simulink model "STATCOM"  (R2024a)
settings: Solver=FixedStepDiscrete  StartTime=0.0  StopTime=0.4  FixedStep=Ts  RelTol=1e-3
InitFcn:
  | Ts=25e-6;
  | xInitial = STATCOMInit;
undefined symbols (not defined in the file or in its folder): DiscIntNeverNeededParam
libraries: spsThreeLevelBridgeLib x4, spsVoltageMeasurementLib x4, spsZigzagPhaseShiftingTransformerLib x4, spsThreePhaseVIMeasurementLib x3, spsDistributedParametersLineLib x3, spsSecondOrderFilterLib x3, spsSeriesRLCBranchLib x2, spsThreePhaseSourceLib x2, spsGroundLib x2, spsabctodq0Lib x2, spsThreePhaseSeriesRLCLoadLib x1, spsThreePhaseParallelRLCLoadLib x1
(part 2 of 3)

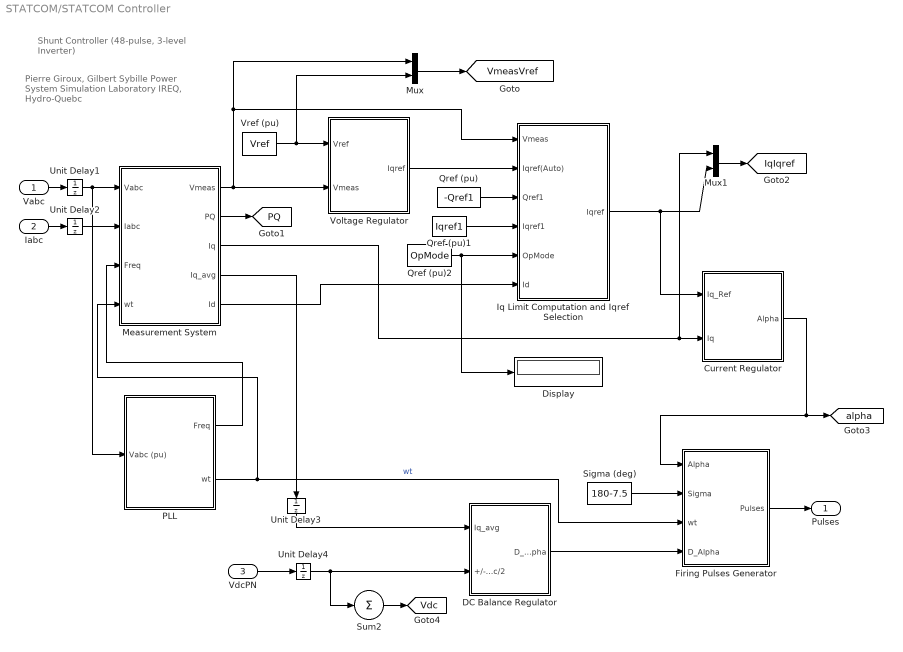
== system STATCOM/STATCOM Controller ==
  note: Pierre Giroux, Gilbert Sybille
      | Power System Simulation Laboratory
      | IREQ, Hydro-Quebc
  note: Shunt Controller
      | (48-pulse, 3-level Inverter)
  Vabc : Inport  PortDimensions=3
  Iabc : Inport  Port=2  PortDimensions=3
  VdcPN : Inport  Port=3  PortDimensions=2
  Current Regulator : Subsystem  mask(Discrete PI Controller){Kp=Kp_I, Ki=Ki_I, Par_Limits=[80 -80], Init=0, Ts=Ts}
      mask prompts: Kp "Proportional gain (Kp):"; Ki "Integral gain (Ki):"; Par_Limits "Output limits: [ Upper   Lower ]"; Init "Output initial value:"; Ts "Sample time:"
      mask help: This block implements a discrete PI controller.
      mask init:
      | UpperLimit=Par_Limits(1);
      | LowerLimit=Par_Limits(2);
  DC Balance Regulator : Subsystem
  Display : Display
  Firing Pulses Generator : Subsystem
  Iq Limit Computation and Iqref Selection : Subsystem
  Measurement System : Subsystem
  Mux : Mux  Inputs=2
  Mux1 : Mux  Inputs=2
  PLL : Subsystem  mask(Discrete 3-phase PLL){Nstep=1, Par_Init=[0 60], ParK=[60 1400], Ts=Ts}
      mask prompts: Nstep "PLL timing correction (in number of time step)"; Par_Init "Initial inputs:[ Phase(degrees)   Frequency(Hz) ]"; ParK "Regulator gains [ Kp  Ki ]"; Ts "Sample time:"
      mask help:
      | This Phase Locked Loop (PLL) system can be used  to synchronize on a set of variable frequency, three-phase sinusoidal signals.
      |
      | Input 1: Vector containing the normalized
      |              three-phase signals [Va Vb Vc]
      | Output 1:  Measured frequency (Hz) = w/(2pi)
      | Output 2:  Ramp w.t   varying between  0 and 2*pi,
      | synchronized on zero crossings of the fundamental (positive-sequence) of phase A.
      | Output 3: Vector [sin(wt) cos(wt)]
      mask init:
      | Kp=ParK(1);
      | Ki=ParK(2);
      | Phase_Init=Par_Init(1);
      | Finit=Par_Init(2);
  Qref (pu) : Constant  Value=-Qref1
  Qref (pu)1 : Constant  Value=Iqref1
  Qref (pu)2 : Constant  Value=OpMode
  Sigma (deg) : Constant  Value=180-7.5
  Sum2 : Sum  Inputs=1  InputSameDT=on  SaturateOnIntegerOverflow=on  OutDataTypeStr=Inherit: Same as first input
  Unit Delay{1..4} (4 alike) : UnitDelay  SampleTime=Ts  HasFrameUpgradeWarning=on
  Voltage Regulator : Subsystem  mask(Discrete PI Controller){Droop=Droop, Kp=Kp_V, Ki=Ki_V, Par_Limits=[1 -1], Init=0, Ts=Ts}
      mask prompts: Droop "Droop (pu/100MVA):"; Kp "Proportional gain (Kp):"; Ki "Integral gain (Ki):"; Par_Limits "Output limits: [ Upper   Lower ]"; Init "Output initial value:"; Ts "Sample time:"
      mask help: This block implements a discrete PI controller.
      mask init:
      | UpperLimit=Par_Limits(1);
      | LowerLimit=Par_Limits(2);
  Vref (pu) : Constant  Value=Vref
  Pulses : Outport  VectorParamsAs1DForOutWhenUnconnected=off
  tag scope: IqIqref=global, PQ=global, Vdc=global, VmeasVref=global, alpha=global
  wires:
  DC Balance Regulator/1(D_Alpha) -> Firing Pulses Generator/4(D_Alpha)
  Unit Delay4/1 -> Sum2/1, DC Balance Regulator/2(+/-Vdc/2)
  Unit Delay2/1 -> Measurement System/2(Iabc)
  Unit Delay1/1 -> Measurement System/1(Vabc), PLL/1(Vabc (pu))
  Sum2/1 -> [Vdc]
  Iabc/1 -> Unit Delay2/1
  Firing Pulses Generator/1(Pulses) -> Pulses/1
  VdcPN/1 -> Unit Delay4/1
  Mux/1 -> [VmeasVref]
  Unit Delay3/1 -> DC Balance Regulator/1(Iq_avg)
  Measurement System/4(Iq_avg) -> Unit Delay3/1
  Vabc/1 -> Unit Delay1/1
  PLL/2(wt) -> Measurement System/4(wt), Firing Pulses Generator/3(wt)  "wt"
  PLL/1(Freq) -> Measurement System/3(Freq)
  Qref (pu)2/1 -> Display/1, Iq Limit Computation and Iqref Selection/5(OpMode)
  Voltage Regulator/1(Iqref) -> Iq Limit Computation and Iqref Selection/2(Iqref(Auto))
  Measurement System/2(PQ) -> [PQ]
  Measurement System/1(Vmeas) -> Mux/1, Iq Limit Computation and Iqref Selection/1(Vmeas), Voltage Regulator/2(Vmeas)
  Qref (pu)/1 -> Iq Limit Computation and Iqref Selection/3(Qref1)
  Qref (pu)1/1 -> Iq Limit Computation and Iqref Selection/4(Iqref1)
  Measurement System/3(Iq) -> Current Regulator/2(Iq), Mux1/1
  Measurement System/5(Id) -> Iq Limit Computation and Iqref Selection/6(Id)
  Vref (pu)/1 -> Voltage Regulator/1(Vref), Mux/2
  Iq Limit Computation and Iqref Selection/1(Iqref) -> Current Regulator/1(Iq_Ref), Mux1/2
  Mux1/1 -> [IqIqref]
  Sigma (deg)/1 -> Firing Pulses Generator/2(Sigma)
  Current Regulator/1(Alpha) -> Firing Pulses Generator/1(Alpha), [alpha]

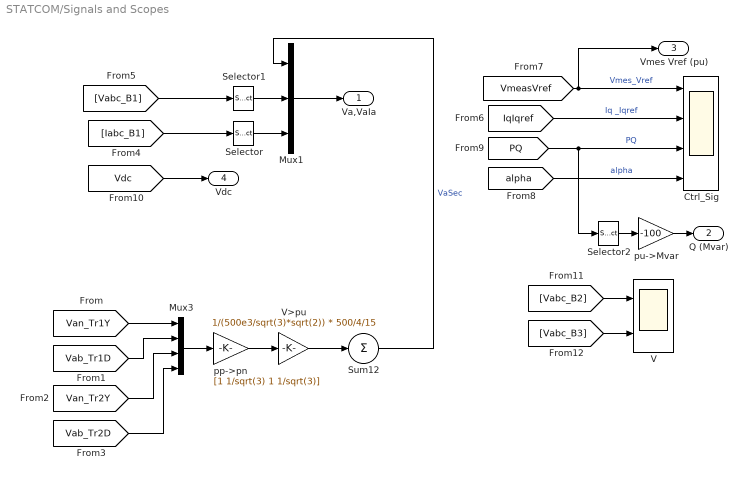
== system STATCOM/Signals and Scopes ==
  Ctrl_Sig : Scope  NumInputPorts=4
  Mux1 : Mux  Inputs=3
  Mux3 : Mux
  Selector : Selector  InputPortWidth=3  IndexOptions=Index vector (dialog)  Indices=1  OutputSizes=1
  Selector1 : Selector  InputPortWidth=3  IndexOptions=Index vector (dialog)  Indices=1  OutputSizes=1
  Selector2 : Selector  InputPortWidth=2  IndexOptions=Index vector (dialog)  Indices=2  OutputSizes=1
  Sum12 : Sum  Inputs=1  InputSameDT=on  SaturateOnIntegerOverflow=on  OutDataTypeStr=Inherit: Same as first input
  V : Scope  NumInputPorts=2
  "V>pu " : Gain  Gain=1/(500e3/sqrt(3)*sqrt(2)) * 500/4/15  SaturateOnIntegerOverflow=on  OutDataTypeStr=Inherit: Same as input  ParamDataTypeStr=Inherit: Same as input
  pp->pn : Gain  Gain=[1 1/sqrt(3) 1 1/sqrt(3)]  SaturateOnIntegerOverflow=on  OutDataTypeStr=Inherit: Same as input  ParamDataTypeStr=Inherit: Same as input
  pu->Mvar : Gain  Gain=-100  SaturateOnIntegerOverflow=on  OutDataTypeStr=Inherit: Same as input  ParamDataTypeStr=Inherit: Same as input
  Va,VaIa : Outport  VectorParamsAs1DForOutWhenUnconnected=off
  "Q (Mvar) " : Outport  Port=2  VectorParamsAs1DForOutWhenUnconnected=off
  Vmes Vref (pu) : Outport  Port=3  VectorParamsAs1DForOutWhenUnconnected=off
  Vdc : Outport  Port=4  VectorParamsAs1DForOutWhenUnconnected=off
  wires:
  "V>pu "/1 -> Sum12/1
  pp->pn/1 -> "V>pu "/1
  Mux3/1 -> pp->pn/1
  [Van_Tr1Y] -> Mux3/1
  [Vab_Tr1D] -> Mux3/2
  [Van_Tr2Y] -> Mux3/3
  [Vab_Tr2D] -> Mux3/4
  Mux1/1 -> Va,VaIa/1
  [VmeasVref] -> Vmes Vref (pu)/1, Ctrl_Sig/1  "Vmes_Vref"
  Selector1/1 -> Mux1/2
  Selector/1 -> Mux1/3
  Sum12/1 -> Mux1/1  "VaSec"
  [IqIqref] -> Ctrl_Sig/2  "Iq _Iqref"
  [PQ] -> Ctrl_Sig/3, Selector2/1  "PQ"
  [alpha] -> Ctrl_Sig/4  "alpha"
  [Vabc_B1] -> Selector1/1
  [Iabc_B1] -> Selector/1
  [Vdc] -> Vdc/1
  [Vabc_B2] -> V/1
  [Vabc_B3] -> V/2
  Selector2/1 -> pu->Mvar/1
  pu->Mvar/1 -> "Q (Mvar) "/1

== system STATCOM/STATCOM Controller/Current Regulator ==
  Iq_Ref : Inport
  Iq : Inport  Port=2
  Discrete-Time Integrator : DiscreteIntegrator  InitialCondition=Init  SampleTime=Ts  LimitOutput=on  UpperSaturationLimit=UpperLimit*10  LowerSaturationLimit=LowerLimit*10  ICPrevOutput=DiscIntNeverNeededParam  ICPrevScaledInput=DiscIntNeverNeededParam
  Kp4 : Gain  Gain=Kp  SaturateOnIntegerOverflow=on  OutDataTypeStr=Inherit: Same as input  ParamDataTypeStr=Inherit: Same as input
  Kp5 : Gain  Gain=Ki  SaturateOnIntegerOverflow=on  OutDataTypeStr=Inherit: Same as input  ParamDataTypeStr=Inherit: Same as input
  Saturation2 : Saturate  UpperLimit=UpperLimit  LowerLimit=LowerLimit
  Sum : Sum  Inputs=-+|  InputSameDT=on  SaturateOnIntegerOverflow=on  OutDataTypeStr=Inherit: Same as first input
  Sum6 : Sum  InputSameDT=on  SaturateOnIntegerOverflow=on  OutDataTypeStr=Inherit: Same as first input
  Alpha : Outport  InitialOutput=0  VectorParamsAs1DForOutWhenUnconnected=off
  wires:
  Sum/1 -> Kp4/1, Kp5/1  "Err"
  Iq/1 -> Sum/2
  Saturation2/1 -> Alpha/1
  Discrete-Time Integrator/1 -> Sum6/2
  Kp4/1 -> Sum6/1
  Kp5/1 -> Discrete-Time Integrator/1
  Sum6/1 -> Saturation2/1
  Iq_Ref/1 -> Sum/1

== system STATCOM/STATCOM Controller/DC Balance Regulator ==
  Iq_avg : Inport  PortDimensions=1
  +/-Vdc/2 : Inport  Port=2  PortDimensions=2
  " Mean value" : Subsystem  mask(Discrete Mean value){Freq=60, Vinit=0, Ts=Ts}
      mask prompts: Freq "Fundamental frequency (Hz):"; Vinit "Initial input (DC component):"; Ts "Sample time:"
      mask help:
      | This block computes the mean value of the input signal over a running window of one cycle of the specified fundamental frequency.
      | For the first cycle of simulation, the output is held constant to the value specified by the parameter "Initial input".
      mask init:
      | SamplesPerCycle=1/Freq/Ts;
      | RoundSamplesPerCycle=round(SamplesPerCycle);
      | Delay=RoundSamplesPerCycle*Ts - Ts/2;
      | Correction=SamplesPerCycle/RoundSamplesPerCycle - 1;
  Abs : Abs
  D_Alpha(Manual) : Constant  Value=0
  D_Alpha1 : Constant  Value=0
  D_Alpha2 : Constant  Value=0
  D_Alpha5 : Constant  Value=0.1
  Demux : Demux  Outputs=2
      settings: DisplayOption=none
  Gain : Gain  Gain=0  SaturateOnIntegerOverflow=on  OutDataTypeStr=Inherit: Same as input  ParamDataTypeStr=Inherit: Same as input
  Gain1 : Gain  Gain=-1  SaturateOnIntegerOverflow=on  OutDataTypeStr=Inherit: Same as input  ParamDataTypeStr=Inherit: Same as input
  Mode : Constant
  Multiport Switch : MultiPortSwitch
  PI Regulator : Subsystem  mask(Discrete PI Controller){Kp=0.001, Ki=0.01, Par_Limits=[2 -2], Init=0, Ts=Ts}
      mask prompts: Kp "Proportional gain (Kp):"; Ki "Integral gain (Ki):"; Par_Limits "Output limits: [ Upper   Lower ]"; Init "Output initial value:"; Ts "Sample time:"
      mask help: This block implements a discrete PI controller.
      mask init:
      | UpperLimit=Par_Limits(1);
      | LowerLimit=Par_Limits(2);
      mask Display: disp('PI');
  Relational Operator : RelationalOperator  Operator=<=
  Relational Operator1 : RelationalOperator  Operator=<
  Sum2 : Sum  Inputs=-+  InputSameDT=on  SaturateOnIntegerOverflow=on  OutDataTypeStr=Inherit: Same as first input
  Switch : Switch  Threshold=0.5
  Switch1 : Switch  Threshold=0.5
  D_Alpha : Outport  VectorParamsAs1DForOutWhenUnconnected=off
  wires:
  Demux/2 -> Sum2/2
  Demux/1 -> Sum2/1
  +/-Vdc/2/1 -> Demux/1
  Iq_avg/1 -> Relational Operator/1, Abs/1
  Sum2/1 -> " Mean value"/1(In)
  Switch1/1 -> PI Regulator/1(Error)
  Gain/1 -> Switch1/1
  " Mean value"/1(Mean) -> Gain/1, Switch1/3
  D_Alpha1/1 -> Relational Operator/2
  Abs/1 -> Relational Operator1/1
  D_Alpha5/1 -> Relational Operator1/2
  Gain1/1 -> Switch/3
  Relational Operator/1 -> Switch/2
  Switch/1 -> Multiport Switch/2  "Auto"
  D_Alpha2/1 -> Multiport Switch/4  "Off"
  Mode/1 -> Multiport Switch/1
  PI Regulator/1(Out) -> Switch/1, Gain1/1
  D_Alpha(Manual)/1 -> Multiport Switch/3  "Man"
  Multiport Switch/1 -> D_Alpha/1
  Relational Operator1/1 -> Switch1/2, PI Regulator/2(Reset)

== system STATCOM/STATCOM Controller/Firing Pulses Generator ==
  Alpha : Inport  PortDimensions=1
  Sigma : Inport  Port=2  PortDimensions=1
  wt : Inport  Port=3  PortDimensions=1
  D_Alpha : Inport  Port=4  PortDimensions=1
  " Deg->Rad" : Gain  Gain=pi/180  SaturateOnIntegerOverflow=on  OutDataTypeStr=Inherit: Same as input  ParamDataTypeStr=Inherit: Same as input
  Bridge 1D : Subsystem
  "Bridge 1Y " : Subsystem
  Bridge 2D : Subsystem
  Bridge 2Y : Subsystem
  Constant : Constant  Value=[0 -30 -15 -45]*pi/180 + 7.5*pi/180
  Deg->Rad : Gain  Gain=pi/180  SaturateOnIntegerOverflow=on  OutDataTypeStr=Inherit: Same as input  ParamDataTypeStr=Inherit: Same as input
  "Deg->Rad " : Gain  Gain=pi/180  SaturateOnIntegerOverflow=on  OutDataTypeStr=Inherit: Same as input  ParamDataTypeStr=Inherit: Same as input
  Demux : Demux
      settings: DisplayOption=none
  Mux : Mux  Inputs=[12 12 12 12]
  Sum : Sum  InputSameDT=on  SaturateOnIntegerOverflow=on  OutDataTypeStr=Inherit: Same as first input
  Pulses : Outport  VectorParamsAs1DForOutWhenUnconnected=off
  wires:
  Alpha/1 -> Deg->Rad/1
  Constant/1 -> Sum/2
  Sum/1 -> Demux/1
  "Bridge 1Y "/1(Pulses) -> Mux/1
  Mux/1 -> Pulses/1
  Demux/1 -> "Bridge 1Y "/1(wt)
  Sigma/1 -> "Deg->Rad "/1
  Demux/2 -> Bridge 1D/1(wt)
  Demux/3 -> Bridge 2Y/1(wt)
  Demux/4 -> Bridge 2D/1(wt)
  Deg->Rad/1 -> "Bridge 1Y "/2(Alpha), Bridge 1D/2(Alpha), Bridge 2Y/2(Alpha), Bridge 2D/2(Alpha)
  "Deg->Rad "/1 -> "Bridge 1Y "/3(Sigma), Bridge 1D/3(Sigma), Bridge 2Y/3(Sigma), Bridge 2D/3(Sigma)
  " Deg->Rad"/1 -> Bridge 2D/4(D_Alpha), Bridge 2Y/4(D_Alpha), Bridge 1D/4(D_Alpha), "Bridge 1Y "/4(D_Alpha)
  D_Alpha/1 -> " Deg->Rad"/1
  Bridge 1D/1(Pulses) -> Mux/2
  Bridge 2Y/1(Pulses) -> Mux/3
  Bridge 2D/1(Pulses) -> Mux/4
  wt/1 -> Sum/1

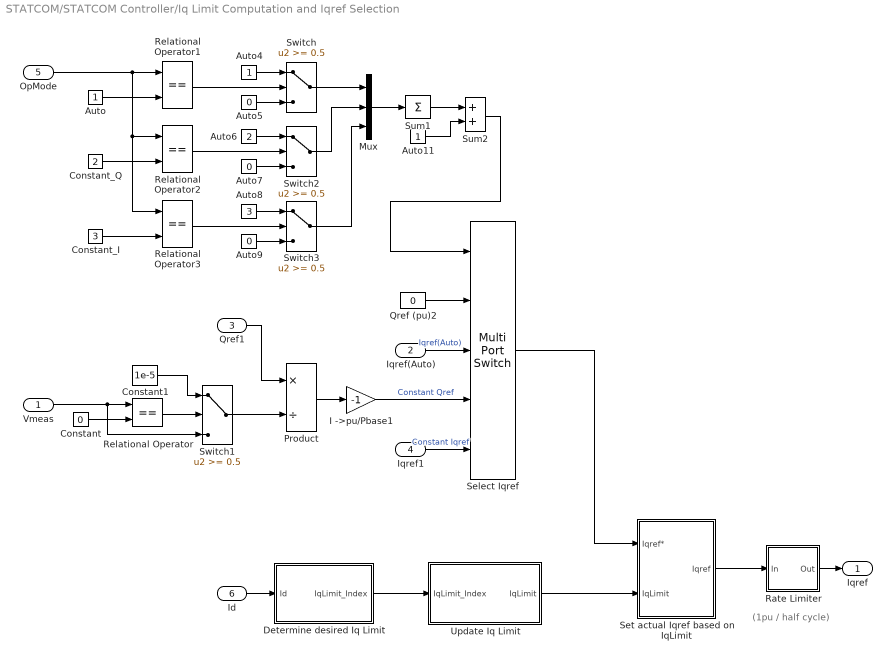
== system STATCOM/STATCOM Controller/Iq Limit Computation and Iqref Selection ==
  note: (1pu / half cycle)
  Vmeas : Inport
  Iqref(Auto) : Inport  Port=2
  Qref1 : Inport  Port=3
  Iqref1 : Inport  Port=4
  OpMode : Inport  Port=5
  Id : Inport  Port=6
  Auto : Constant
  Auto11 : Constant
  Auto4 : Constant
  Auto5 : Constant  Value=0
  Auto6 : Constant  Value=2
  Auto7 : Constant  Value=0
  Auto8 : Constant  Value=3
  Auto9 : Constant  Value=0
  Constant : Constant  Value=0
  Constant1 : Constant  Value=1e-5
  Constant_I : Constant  Value=3
  Constant_Q : Constant  Value=2
  Determine desired Iq Limit : Subsystem
  I ->pu/Pbase1 : Gain  Gain=-1  SaturateOnIntegerOverflow=on  OutDataTypeStr=Inherit: Same as input  ParamDataTypeStr=Inherit: Same as input
  Mux : Mux  Inputs=3
  Product : Product  Inputs=*/  InputSameDT=on  SaturateOnIntegerOverflow=on  OutDataTypeStr=Inherit: Same as first input
  Qref (pu)2 : Constant  Value=0
  "Rate Limiter " : Subsystem  DialogController=POWERSYS.PowerSysDialog  mask(Discrete Rate Limiter){R=120, F=-120, Vinit=-0.33, Ts=Ts}
      mask prompts: R "Rising slew rate:"; F "Falling slew rate:"; Vinit "Initial input:"; Ts "Sample time:"
      mask help: DISCRETE BLOCK : Limit rising and falling rates of signal
      mask init:
      | UpperLimit=R*Ts;
      | LowerLimit=F*Ts;
      | power_initmask();
      mask Help: This block is part of a subset of blocks in the Extras library that does not have documentation associated with it, other than the block mask description.
      mask Display: disp('Discrete\nRate\nLimiter')
  Relational Operator{,1..3} (4 alike) : RelationalOperator  Operator===
  Select Iqref : MultiPortSwitch  Inputs=4
  Set actual Iqref based on IqLimit : Subsystem
  Sum1 : Sum  Inputs=1  InputSameDT=on  SaturateOnIntegerOverflow=on  OutDataTypeStr=Inherit: Same as first input
  Sum2 : Sum  InputSameDT=on  SaturateOnIntegerOverflow=on  OutDataTypeStr=Inherit: Same as first input
  Switch{,1..3} (4 alike) : Switch  Threshold=0.5
  Update Iq Limit : Subsystem
  Iqref : Outport  VectorParamsAs1DForOutWhenUnconnected=off
  wires:
  Set actual Iqref based on IqLimit/1(Iqref) -> "Rate Limiter "/1(In)
  Switch2/1 -> Mux/2
  Auto11/1 -> Sum2/2
  Sum1/1 -> Sum2/1
  Switch3/1 -> Mux/3
  Mux/1 -> Sum1/1
  Switch/1 -> Mux/1
  Auto9/1 -> Switch3/3
  Auto8/1 -> Switch3/1
  Relational Operator3/1 -> Switch3/2
  Auto7/1 -> Switch2/3
  Auto6/1 -> Switch2/1
  Relational Operator2/1 -> Switch2/2
  Auto5/1 -> Switch/3
  Auto4/1 -> Switch/1
  Relational Operator1/1 -> Switch/2
  OpMode/1 -> Relational Operator3/1, Relational Operator2/1, Relational Operator1/1
  Constant_I/1 -> Relational Operator3/2
  Constant_Q/1 -> Relational Operator2/2
  Auto/1 -> Relational Operator1/2
  Sum2/1 -> Select Iqref/1
  Vmeas/1 -> Relational Operator/1, Switch1/3
  Qref1/1 -> Product/1
  Relational Operator/1 -> Switch1/2
  Constant1/1 -> Switch1/1
  Switch1/1 -> Product/2
  Constant/1 -> Relational Operator/2
  Product/1 -> I ->pu/Pbase1/1
  Iqref1/1 -> Select Iqref/5  "Constant Iqref"
  Iqref(Auto)/1 -> Select Iqref/3  "Iqref(Auto)"
  I ->pu/Pbase1/1 -> Select Iqref/4  "Constant Qref"
  Qref (pu)2/1 -> Select Iqref/2
  Select Iqref/1 -> Set actual Iqref based on IqLimit/1(Iqref*)
  Determine desired Iq Limit/1(IqLimit_Index) -> Update Iq Limit/1(IqLimit_Index)
  Update Iq Limit/1(IqLimit) -> Set actual Iqref based on IqLimit/2(IqLimit)
  "Rate Limiter "/1(Out) -> Iqref/1
  Id/1 -> Determine desired Iq Limit/1(Id)

== system STATCOM/STATCOM Controller/Measurement System ==
  Vabc : Inport  PortDimensions=3
  Iabc : Inport  Port=2  PortDimensions=3
  Freq : Inport  Port=3  PortDimensions=1
  wt : Inport  Port=4  PortDimensions=1
  Mean value : Subsystem  mask(Discrete Variable-Frequency Mean Value){Finit=60, Vinit=0, Ts=Ts}
      mask prompts: Finit "Initial Frequency (Hz):"; Vinit "Initial input (DC component):"; Ts "Sample time:"
      mask help:
      | This discrete block computes the mean value of the input signal (port In) over a running window of one cycle of a specified frequency (port Freq).
      |
      | For the first cycle of simulation (specified by the parameter "Initial frequency"), the output is held to the value of the  "Initial input" parameter.
  Mux : Mux  Inputs=2
  PQ Computaion : Subsystem
  Reactive current measurement (Iq) : Subsystem  mask(abc to dq0 Transformation){}
      mask help:
      | This block performs the  abc to dq0 transformation on a set of three-phase signals.
      |
      | It computes the three components ( Vd=direct axis , Vq=quadrature axis and V0=zero sequence) in a two axis rotating reference frame according to the following transformation:
      |
      | Vd = 2/3*[Va*sin(wt)  + Vb*sin(wt-2pi/3)  +  Vc*sin(wt+2pi/3)]
      | Vq = 2/3*[Va*cos(wt) + Vb*cos(wt-2pi/3) + Vc*cos(wt+2pi/3)]
      | V0 = 1/3*[Va +  Vb  +  Vc ]
      | where w=  rotation speed (rad/s) of the rotating frame.
      |
      | Input 1 contains  the vectorized  signals of the three  [Va Vb  Vc] sinusoidal phase quantities.
      | Input 2 must contain a  [sin(wt)  cos(wt)] two dimension signal , where w is the rotation speed (rad/s)  of the reference frame.
      | Output is a vectozized signal containing the [Vd Vq Vo] components.
      |
      | Press Help for more information.
      mask Help:
      | This transformation is commonly used in three-phase electric machine models where it is known as Park transformation. It allows to eliminate time varying inductances by referring the stator and rotor quantities to a fixed or rotating reference frame .
      | In case of a synchrounous machine, the stator quantities are referred to the rotor. Id and Iq represent the two DC currents flowing  in the two equivalent rotor windings ( d winding on the same axis as the field winding, and q winding in quadrature) producing the same flux as the stator Ia, Ib and Ic currents.
      | 
      | You can also use this block in a control system to measure the positive-sequence component V1 of a set of three-phase voltages or currents.
      | Vd and Vq represent the rectangular coordinates of  V1.
      | Use the Math Function block (hypot) and the Trigonometric function block (atan2) to obtain the modulus and angle of V1.
      | Mag(V1) = sqrt(Vd^2 + Vq^2);
      | Phase(V1)=atan2(Vq/Vd).
      | This measurement system does not introduce any delay, but, in contrast with the Fourier analysis (See Sequence Analyzer block), it is sensitive to harmonics and unbalances.
      | 
      | See also the dq0_to_abc block performing the reverse transformation.
  Second-Order Filter : spsSecondOrderFilterLib/Second-Order Filter  FilterType=Lowpass  Fo=1200  Zeta=0.707  Ts=Ts  Initialize=off  Vac_Init="[0,  0,  60]"  Vdc_Init=0  PlotResponse=off  FreqRange=[0, 500, 1]
  Second-Order Filter1 : spsSecondOrderFilterLib/Second-Order Filter  FilterType=Lowpass  Fo=1200  Zeta=0.707  Ts=Ts  Initialize=off  Vac_Init="[0,  0,  60]"  Vdc_Init=0  PlotResponse=off  FreqRange=[0, 500, 1]
  Selector : Selector  InputPortWidth=2  IndexOptions=Index vector (dialog)  Indices=2  OutputSizes=1
  Selector1 : Selector  InputPortWidth=2  IndexOptions=Index vector (dialog)  Indices=1  OutputSizes=1
  Trigonometric Function : Trigonometry
  Trigonometric Function1 : Trigonometry  Operator=cos
  Voltage measurement (Positive sequence) : Subsystem  mask(Discrete 3-phase PLL-Driven Positive-Sequence Fundamental Value){Finit=60, Par_Init=[1 0], Ts=Ts}
      mask prompts: Finit "Initial fundamental frequency (Hz):"; Par_Init "Initial input (positive component): [ Mag  Phase-relative-to-PLL(degrees) ]"; Ts "Sample time:"
      mask help:
      | For a supplied fundamental frequency (port Freq), this discrete block computes  the positive-sequence component (Magnitude and Phase)  of a set of three balanced or unbalanced signals (port abc) which may contain harmonics.
      |  Input port "Sin_Cos" (a two-dimension signal) provides the reference frame required for the computation..
      |  First and second outputs return respectively the magnitude and phase (in degrees relative to the PLL phase)) of the fundamental.
      | For the first cycle of simulation, the outputs are held constant to the values specified by the parameter "Initial input".
      mask init:
      | Real_Init=Par_Init(1)*cos(pi/180*Par_Init(2));
      | Imag_Init=Par_Init(1)*sin(pi/180*Par_Init(2));
  Vmeas : Outport  VectorParamsAs1DForOutWhenUnconnected=off
  PQ : Outport  Port=2  VectorParamsAs1DForOutWhenUnconnected=off
  Iq : Outport  Port=3  VectorParamsAs1DForOutWhenUnconnected=off
  Iq_avg : Outport  Port=4  VectorParamsAs1DForOutWhenUnconnected=off
  Id : Outport  Port=5  VectorParamsAs1DForOutWhenUnconnected=off
  wires:
  Second-Order Filter/1 -> Id/1
  Selector1/1 -> Second-Order Filter/1
  Mean value/1(Mean) -> Iq_avg/1
  Selector/1 -> Second-Order Filter1/1, Mean value/2(In)
  Freq/1 -> Mean value/1(Freq), PQ Computaion/3(Freq), Voltage measurement (Positive sequence)/2(Freq)
  Reactive current measurement (Iq)/1(IdIq) -> Selector1/1, Selector/1, PQ Computaion/2(Id_Iq)
  PQ Computaion/1(PQ(pu)) -> PQ/1
  Mux/1 -> Reactive current measurement (Iq)/1(sin_cos)
  Iabc/1 -> Reactive current measurement (Iq)/2(abc)
  wt/1 -> Voltage measurement (Positive sequence)/3(wt), Trigonometric Function1/1, Trigonometric Function/1
  Trigonometric Function1/1 -> Mux/2
  Trigonometric Function/1 -> Mux/1
  Vabc/1 -> Voltage measurement (Positive sequence)/1(abc)
  Voltage measurement (Positive sequence)/1(Mag) -> Vmeas/1  "Vmes"
  Voltage measurement (Positive sequence)/2(VdVq) -> PQ Computaion/1(Vd_Vq)
  Second-Order Filter1/1 -> Iq/1

== system STATCOM/STATCOM Controller/PLL ==
  Vabc (pu) : Inport  PortDimensions=3
  Constant4 : Constant  Value=2*pi
  Correction for delay : Gain  Gain=Nstep*Ts*2*pi  SaturateOnIntegerOverflow=on  OutDataTypeStr=Inherit: Same as input  ParamDataTypeStr=Inherit: Same as input
  Discrete PI Controller : Subsystem  DialogController=POWERSYS.PowerSysDialog  mask(Discrete PI Controller){Kp=Kp, Ki=Ki, Par_Limits=2*pi*Finit*[1.25 0.75], Init=2*pi*Finit, Ts=Ts}
      mask prompts: Kp "Proportional gain (Kp):"; Ki "Integral gain (Ki):"; Par_Limits "Output limits: [ Upper   Lower ]"; Init "Output initial value:"; Ts "Sample time:"
      mask help: This block implements a discrete PI controller.
      mask init:
      | UpperLimit=Par_Limits(1);
      | LowerLimit=Par_Limits(2);
      | power_initmask();
      mask Help: This block is part of a subset of blocks in the Extras library that does not have documentation associated with it, other than the block mask description.
      mask Display: disp('PI');
  Discrete Rate Limiter : Subsystem  DialogController=POWERSYS.PowerSysDialog  mask(Discrete Rate Limiter){R=10, F=-10, Vinit=Finit, Ts=Ts}
      mask prompts: R "Rising slew rate:"; F "Falling slew rate:"; Vinit "Initial input:"; Ts "Sample time:"
      mask help: DISCRETE BLOCK : Limit rising and falling rates of signal
      mask init:
      | UpperLimit=R*Ts;
      | LowerLimit=F*Ts;
      | power_initmask();
      mask Help: This block is part of a subset of blocks in the Extras library that does not have documentation associated with it, other than the block mask description.
      mask Display: disp('Discrete\nRate\nLimiter')
  Discrete-Time Integrator : DiscreteIntegrator  InitialCondition=Phase_Init*pi/180  SampleTime=Ts  ICPrevOutput=DiscIntNeverNeededParam  ICPrevScaledInput=DiscIntNeverNeededParam
  Gain10 : Gain  Gain=1/2/pi  SaturateOnIntegerOverflow=on  OutDataTypeStr=Inherit: Same as input  ParamDataTypeStr=Inherit: Same as input
  Math Function : Math  Operator=mod  SignedPower=on
  Mean (Variable Frequency) : spsMeanVariableFrequencyLib/Mean (Variable Frequency)  Finit=Finit  Fmin=45  Vinit=0  Ts=Ts
  Second-Order Filter : spsSecondOrderFilterLib/Second-Order Filter  FilterType=Lowpass  Fo=25  Zeta=0.707  Ts=Ts  Initialize=on  Vac_Init=[0 -25 60]  Vdc_Init=Finit  PlotResponse=off  FreqRange=[0, 500, 1]
  Selector : Selector  InputPortWidth=3  IndexOptions=Index vector (dialog)  Indices=2  OutputSizes=1
  Sum : Sum  InputSameDT=on  SaturateOnIntegerOverflow=on  OutDataTypeStr=Inherit: Same as first input
  Unit Delay : UnitDelay  InitialCondition=Finit  SampleTime=Ts  HasFrameUpgradeWarning=on
  abc to dq0 : spsabctodq0Lib/abc to dq0  Alignment=90 degrees behind phase A axis
  Freq : Outport  VectorParamsAs1DForOutWhenUnconnected=off
  wt : Outport  Port=2  VectorParamsAs1DForOutWhenUnconnected=off
  wires:
  Sum/1 -> wt/1
  Selector/1 -> Mean (Variable Frequency)/2  "Vq"
  Second-Order Filter/1 -> Unit Delay/1
  Unit Delay/1 -> Correction for delay/1, Mean (Variable Frequency)/1, Freq/1
  Discrete Rate Limiter/1(Out) -> Second-Order Filter/1
  Gain10/1 -> Discrete Rate Limiter/1(In)
  Discrete PI Controller/1(Out) -> Gain10/1, Discrete-Time Integrator/1  "W"
  Math Function/1 -> abc to dq0/2, Sum/2
  Discrete-Time Integrator/1 -> Math Function/1
  Constant4/1 -> Math Function/2
  abc to dq0/1 -> Selector/1
  Vabc (pu)/1 -> abc to dq0/1
  Mean (Variable Frequency)/1 -> Discrete PI Controller/1(Error)
  Correction for delay/1 -> Sum/1

== system STATCOM/STATCOM Controller/Voltage Regulator ==
  Vref : Inport
  Vmeas : Inport  Port=2
  Discrete-Time Integrator : DiscreteIntegrator  InitialCondition=Init  SampleTime=Ts  LimitOutput=on  UpperSaturationLimit=UpperLimit  LowerSaturationLimit=LowerLimit  ICPrevOutput=DiscIntNeverNeededParam  ICPrevScaledInput=DiscIntNeverNeededParam
  Kp4 : Gain  Gain=Kp  SaturateOnIntegerOverflow=on  OutDataTypeStr=Inherit: Same as input  ParamDataTypeStr=Inherit: Same as input
  Kp5 : Gain  Gain=Ki  SaturateOnIntegerOverflow=on  OutDataTypeStr=Inherit: Same as input  ParamDataTypeStr=Inherit: Same as input
  Kp6 : Gain  Gain=Droop  SaturateOnIntegerOverflow=on  OutDataTypeStr=Inherit: Same as input  ParamDataTypeStr=Inherit: Same as input
  Saturation2 : Saturate  UpperLimit=UpperLimit  LowerLimit=LowerLimit
  Sum1 : Sum  Inputs=|-+  InputSameDT=on  SaturateOnIntegerOverflow=on  OutDataTypeStr=Inherit: Same as first input
  Sum6 : Sum  InputSameDT=on  SaturateOnIntegerOverflow=on  OutDataTypeStr=Inherit: Same as first input
  Sum7 : Sum  Inputs=|+-  InputSameDT=on  SaturateOnIntegerOverflow=on  OutDataTypeStr=Inherit: Same as first input
  Unit Delay : UnitDelay  SampleTime=Ts  HasFrameUpgradeWarning=on
  Iqref : Outport  InitialOutput=0  VectorParamsAs1DForOutWhenUnconnected=off
  wires:
  Sum1/1 -> Sum7/1  "Err"
  Vref/1 -> Sum1/2
  Vmeas/1 -> Sum1/1
  Unit Delay/1 -> Sum7/2
  Kp6/1 -> Unit Delay/1
  Saturation2/1 -> Kp6/1, Iqref/1  "Iq_Ref"
  Sum7/1 -> Kp4/1, Kp5/1
  Kp5/1 -> Discrete-Time Integrator/1
  Sum6/1 -> Saturation2/1
  Kp4/1 -> Sum6/1
  Discrete-Time Integrator/1 -> Sum6/2

== system STATCOM/STATCOM Controller/DC Balance Regulator/ Mean value ==
  note: Pierre Giroux, Gilbert Sybille
      | Power System Simulation Laboratory
      | IREQ, Hydro-Quebc
  note: Discrete Mean Value
  In : Inport
  Constant : Constant  Value=Vinit
  Constant1 : Constant  Value=Correction
  Integ4 : DiscreteIntegrator  IntegratorMethod=Integration: Trapezoidal  SampleTime=Ts  ICPrevOutput=DiscIntNeverNeededParam  ICPrevScaledInput=DiscIntNeverNeededParam
  K2 : Constant  Value=Freq
  Product : Product  InputSameDT=on  SaturateOnIntegerOverflow=on  OutDataTypeStr=Inherit: Same as first input
  Product1 : Product  Inputs=**  InputSameDT=on  SaturateOnIntegerOverflow=on  OutDataTypeStr=Inherit: Same as first input
  Step : Step  Time=1/Freq  SampleTime=Ts
  Sum5 : Sum  InputSameDT=on  SaturateOnIntegerOverflow=on  OutDataTypeStr=Inherit: Same as first input
  Sum7 : Sum  Inputs=-+  InputSameDT=on  SaturateOnIntegerOverflow=on  OutDataTypeStr=Inherit: Same as first input
  Switch : Switch  Threshold=0.5
  Transport Delay : TransportDelay  DelayTime=Delay
  Mean : Outport  VectorParamsAs1DForOutWhenUnconnected=off
  wires:
  Product/1 -> Sum5/1  "Mean value"
  Transport Delay/1 -> Sum7/1
  Sum7/1 -> Product/1
  Integ4/1 -> Transport Delay/1, Sum7/2
  K2/1 -> Product/2
  In/1 -> Integ4/1, Product1/1  "In"
  Constant1/1 -> Product1/2
  Product1/1 -> Sum5/2  "Correction"
  Sum5/1 -> Switch/1
  Step/1 -> Switch/2
  Constant/1 -> Switch/3
  Switch/1 -> Mean/1

== system STATCOM/STATCOM Controller/DC Balance Regulator/PI Regulator ==
  note: Pierre Giroux, Gilbert Sybille
      | Power System Simulation Laboratory
      | IREQ, Hydro-Quebc
  note: Discrete PID Controller
  Error : Inport
  Reset : Inport  Port=2
  Discrete-Time Integrator : DiscreteIntegrator  ExternalReset=rising  InitialCondition=Init  SampleTime=Ts  LimitOutput=on  UpperSaturationLimit=UpperLimit  LowerSaturationLimit=LowerLimit  ICPrevOutput=DiscIntNeverNeededParam  ICPrevScaledInput=DiscIntNeverNeededParam
  Kp4 : Gain  Gain=Kp  SaturateOnIntegerOverflow=on  OutDataTypeStr=Inherit: Same as input  ParamDataTypeStr=Inherit: Same as input
  Kp5 : Gain  Gain=Ki  SaturateOnIntegerOverflow=on  OutDataTypeStr=Inherit: Same as input  ParamDataTypeStr=Inherit: Same as input
  Saturation2 : Saturate  UpperLimit=UpperLimit  LowerLimit=LowerLimit
  Sum6 : Sum  InputSameDT=on  SaturateOnIntegerOverflow=on  OutDataTypeStr=Inherit: Same as first input
  Out : Outport  InitialOutput=0  VectorParamsAs1DForOutWhenUnconnected=off
  wires:
  Saturation2/1 -> Out/1
  Discrete-Time Integrator/1 -> Sum6/2
  Kp4/1 -> Sum6/1
  Kp5/1 -> Discrete-Time Integrator/1
  Sum6/1 -> Saturation2/1
  Error/1 -> Kp5/1, Kp4/1
  Reset/1 -> Discrete-Time Integrator/2

== system STATCOM/STATCOM Controller/Firing Pulses Generator/Bridge 1D ==
  wt : Inport  PortDimensions=1
  Alpha : Inport  Port=2  PortDimensions=1
  Sigma : Inport  Port=3  PortDimensions=1
  D_Alpha : Inport  Port=4  PortDimensions=1
  Constant : Constant  Value=-2*pi/3
  Constant1 : Constant  Value=2*pi/3
  Mux1 : Mux  Inputs=[4 4 4]
  Phase A : Subsystem
  Phase B : Subsystem
  Phase C : Subsystem
  Sum : Sum  InputSameDT=on  SaturateOnIntegerOverflow=on  OutDataTypeStr=Inherit: Same as first input
  Sum1 : Sum  InputSameDT=on  SaturateOnIntegerOverflow=on  OutDataTypeStr=Inherit: Same as first input
  Sum2 : Sum  InputSameDT=on  SaturateOnIntegerOverflow=on  OutDataTypeStr=Inherit: Same as first input
  Pulses : Outport  VectorParamsAs1DForOutWhenUnconnected=off
  wires:
  Constant1/1 -> Sum1/2
  Sigma/1 -> Phase A/2(sigma), Phase C/2(sigma), Phase B/2(sigma)
  Alpha/1 -> Sum2/2
  wt/1 -> Sum2/1
  Sum2/1 -> Phase A/1(wt), Sum/1, Sum1/1
  Mux1/1 -> Pulses/1
  Phase A/1(Pulses) -> Mux1/1
  Constant/1 -> Sum/2
  Sum/1 -> Phase B/1(wt)
  Sum1/1 -> Phase C/1(wt)
  D_Alpha/1 -> Phase A/3(D_Alpha), Phase B/3(D_Alpha), Phase C/3(D_Alpha)
  Phase B/1(Pulses) -> Mux1/2
  Phase C/1(Pulses) -> Mux1/3

== system STATCOM/STATCOM Controller/Firing Pulses Generator/Bridge 1Y  ==
  wt : Inport  PortDimensions=1
  Alpha : Inport  Port=2  PortDimensions=1
  Sigma : Inport  Port=3  PortDimensions=1
  D_Alpha : Inport  Port=4  PortDimensions=1
  Constant : Constant  Value=-2*pi/3
  Constant1 : Constant  Value=2*pi/3
  Mux1 : Mux  Inputs=[4 4 4]
  Phase A : Subsystem
  Phase B : Subsystem
  Phase C : Subsystem
  Sum : Sum  InputSameDT=on  SaturateOnIntegerOverflow=on  OutDataTypeStr=Inherit: Same as first input
  Sum1 : Sum  InputSameDT=on  SaturateOnIntegerOverflow=on  OutDataTypeStr=Inherit: Same as first input
  Sum2 : Sum  InputSameDT=on  SaturateOnIntegerOverflow=on  OutDataTypeStr=Inherit: Same as first input
  Pulses : Outport  VectorParamsAs1DForOutWhenUnconnected=off
  wires:
  Phase C/1(Pulses) -> Mux1/3
  Phase B/1(Pulses) -> Mux1/2
  D_Alpha/1 -> Phase C/3(D_Alpha), Phase B/3(D_Alpha), Phase A/3(D_Alpha)
  Sum1/1 -> Phase C/1(wt)
  Sum/1 -> Phase B/1(wt)
  Constant/1 -> Sum/2
  Phase A/1(Pulses) -> Mux1/1
  Mux1/1 -> Pulses/1
  Sum2/1 -> Sum1/1, Sum/1, Phase A/1(wt)
  wt/1 -> Sum2/1
  Alpha/1 -> Sum2/2
  Sigma/1 -> Phase B/2(sigma), Phase C/2(sigma), Phase A/2(sigma)
  Constant1/1 -> Sum1/2

== system STATCOM/STATCOM Controller/Firing Pulses Generator/Bridge 2D ==
  wt : Inport  PortDimensions=1
  Alpha : Inport  Port=2  PortDimensions=1
  Sigma : Inport  Port=3  PortDimensions=1
  D_Alpha : Inport  Port=4  PortDimensions=1
  Constant : Constant  Value=-2*pi/3
  Constant1 : Constant  Value=2*pi/3
  Mux1 : Mux  Inputs=[4 4 4]
  Phase A : Subsystem
  Phase B : Subsystem
  Phase C : Subsystem
  Sum : Sum  InputSameDT=on  SaturateOnIntegerOverflow=on  OutDataTypeStr=Inherit: Same as first input
  Sum1 : Sum  InputSameDT=on  SaturateOnIntegerOverflow=on  OutDataTypeStr=Inherit: Same as first input
  Sum2 : Sum  InputSameDT=on  SaturateOnIntegerOverflow=on  OutDataTypeStr=Inherit: Same as first input
  Pulses : Outport  VectorParamsAs1DForOutWhenUnconnected=off
  wires:
  Constant1/1 -> Sum1/2
  Sigma/1 -> Phase A/2(sigma), Phase C/2(sigma), Phase B/2(sigma)
  Alpha/1 -> Sum2/2
  wt/1 -> Sum2/1
  Sum2/1 -> Phase A/1(wt), Sum/1, Sum1/1
  Mux1/1 -> Pulses/1
  Phase A/1(Pulses) -> Mux1/1
  Constant/1 -> Sum/2
  Sum/1 -> Phase B/1(wt)
  Sum1/1 -> Phase C/1(wt)
  D_Alpha/1 -> Phase A/3(D_Alpha), Phase B/3(D_Alpha), Phase C/3(D_Alpha)
  Phase B/1(Pulses) -> Mux1/2
  Phase C/1(Pulses) -> Mux1/3

== system STATCOM/STATCOM Controller/Firing Pulses Generator/Bridge 2Y ==
  wt : Inport  PortDimensions=1
  Alpha : Inport  Port=2  PortDimensions=1
  Sigma : Inport  Port=3  PortDimensions=1
  D_Alpha : Inport  Port=4  PortDimensions=1
  Constant : Constant  Value=-2*pi/3
  Constant1 : Constant  Value=2*pi/3
  Mux1 : Mux  Inputs=[4 4 4]
  Phase A : Subsystem
  Phase B : Subsystem
  Phase C : Subsystem
  Sum : Sum  InputSameDT=on  SaturateOnIntegerOverflow=on  OutDataTypeStr=Inherit: Same as first input
  Sum1 : Sum  InputSameDT=on  SaturateOnIntegerOverflow=on  OutDataTypeStr=Inherit: Same as first input
  Sum2 : Sum  InputSameDT=on  SaturateOnIntegerOverflow=on  OutDataTypeStr=Inherit: Same as first input
  Pulses : Outport  VectorParamsAs1DForOutWhenUnconnected=off
  wires:
  Phase C/1(Pulses) -> Mux1/3
  Phase B/1(Pulses) -> Mux1/2
  D_Alpha/1 -> Phase C/3(D_Alpha), Phase B/3(D_Alpha), Phase A/3(D_Alpha)
  Sum1/1 -> Phase C/1(wt)
  Sum/1 -> Phase B/1(wt)
  Constant/1 -> Sum/2
  Phase A/1(Pulses) -> Mux1/1
  Mux1/1 -> Pulses/1
  Sum2/1 -> Sum1/1, Sum/1, Phase A/1(wt)
  wt/1 -> Sum2/1
  Alpha/1 -> Sum2/2
  Sigma/1 -> Phase B/2(sigma), Phase C/2(sigma), Phase A/2(sigma)
  Constant1/1 -> Sum1/2

== system STATCOM/STATCOM Controller/Iq Limit Computation and Iqref Selection/Determine desired Iq Limit ==
  note: Determine desired Iq Limit (by step of 0.1 pu, from 1 to 0.3 pu)
      | based on actual value of Id
      | 5% above rated current is allowed
      | i.e.   sqrt ( Id^2 + Iq^2 ) < 1.05 pu
  Id : Inport  PortDimensions=1
  Abs : Abs
  Constant : Constant
  Limit at 0.3 : Relay  OnSwitchValue=0.97  OffSwitchValue=0.92
  Limit at 0.4 : Relay  OnSwitchValue=0.92  OffSwitchValue=0.86
  Limit at 0.5 : Relay  OnSwitchValue=0.86  OffSwitchValue=0.78
  Limit at 0.6 : Relay  OnSwitchValue=0.78  OffSwitchValue=0.68
  Limit at 0.7 : Relay  OnSwitchValue=0.68  OffSwitchValue=0.54
  Limit at 0.8 : Relay  OnSwitchValue=0.54  OffSwitchValue=0.32
  Limit at 0.9 : Relay  OnSwitchValue=0.32  OffSwitchValue=0.25
  Sum : Sum  Inputs=++++++++  InputSameDT=on  SaturateOnIntegerOverflow=on  OutDataTypeStr=Inherit: Same as first input
  IqLimit_Index : Outport  VectorParamsAs1DForOutWhenUnconnected=off
  wires:
  Limit at 0.3/1 -> Sum/8
  Limit at 0.4/1 -> Sum/7
  Limit at 0.5/1 -> Sum/6
  Abs/1 -> Limit at 0.3/1, Limit at 0.4/1, Limit at 0.5/1, Limit at 0.6/1, Limit at 0.7/1, Limit at 0.8/1, Limit at 0.9/1
  Id/1 -> Abs/1
  Constant/1 -> Sum/1
  Limit at 0.6/1 -> Sum/5
  Limit at 0.7/1 -> Sum/4
  Limit at 0.8/1 -> Sum/3
  Limit at 0.9/1 -> Sum/2
  Sum/1 -> IqLimit_Index/1

== system STATCOM/STATCOM Controller/Iq Limit Computation and Iqref Selection/Rate Limiter  ==
  note: Beat Ronner
      | ABB Industrie AG
      | Turgi, Switzerland
  note: Delta(u)
  In : Inport
  Saturation : Saturate  UpperLimit=UpperLimit  LowerLimit=LowerLimit
  Sum : Sum  Inputs=|++  InputSameDT=on  SaturateOnIntegerOverflow=on  OutDataTypeStr=Inherit: Same as first input
  Sum1 : Sum  Inputs=|+-  InputSameDT=on  SaturateOnIntegerOverflow=on  OutDataTypeStr=Inherit: Same as first input
  Unit Delay : UnitDelay  InitialCondition=Vinit  SampleTime=Ts  HasFrameUpgradeWarning=on
  Out : Outport  VectorParamsAs1DForOutWhenUnconnected=off
  wires:
  Unit Delay/1 -> Sum/2, Sum1/2  "y-1"
  Sum/1 -> Unit Delay/1, Out/1  "y"
  Saturation/1 -> Sum/1  "Delta(u)_limit"
  Sum1/1 -> Saturation/1
  In/1 -> Sum1/1  "u"

== system STATCOM/STATCOM Controller/Iq Limit Computation and Iqref Selection/Set actual Iqref based on IqLimit ==
  Iqref* : Inport  PortDimensions=1
  IqLimit : Inport  Port=2
  Gain2 : Gain  Gain=-1  SaturateOnIntegerOverflow=on  OutDataTypeStr=Inherit: Same as input  ParamDataTypeStr=Inherit: Same as input
  Logical Operator : Logic  Operator=OR
  Product : Product  InputSameDT=on  SaturateOnIntegerOverflow=on  OutDataTypeStr=Inherit: Same as first input
  Relational Operator1 : RelationalOperator  Operator=>
  Relational Operator2 : RelationalOperator  Operator=<
  Sign : Signum
  Switch1 : Switch  Threshold=0.5
  Iqref : Outport  VectorParamsAs1DForOutWhenUnconnected=off
  wires:
  Product/1 -> Switch1/1
  Sign/1 -> Product/2
  Iqref*/1 -> Sign/1, Switch1/3, Relational Operator2/1, Relational Operator1/1
  Logical Operator/1 -> Switch1/2
  Relational Operator2/1 -> Logical Operator/2
  Relational Operator1/1 -> Logical Operator/1
  Gain2/1 -> Relational Operator2/2
  IqLimit/1 -> Gain2/1, Relational Operator1/2, Product/1
  Switch1/1 -> Iqref/1

== system STATCOM/STATCOM Controller/Iq Limit Computation and Iqref Selection/Update Iq Limit ==
  note: 1) Instantaneous update of IqLimit if the new desired Iq limit is lower then the actual limit
  note: Rules for updating the Iq Limit in order to avoid control instability :
  note: 2) Update of the new desired Iq limit is delayed by 3 cycles if the new desired limit is higher then the actual limit
  IqLimit_Index : Inport
  Constant1 : Constant  Value=0.8
  Constant10 : Constant  Value=-1e6
  Constant11 : Constant  Value=3
  Constant2 : Constant  Value=0.7
  Constant3 : Constant  Value=0.6
  Constant4 : Constant  Value=0.5
  Constant5 : Constant  Value=0.4
  Constant6 : Constant
  Constant7 : Constant  Value=0.9
  Constant8 : Constant  Value=0.3
  Constant9 : Constant  Value=60
  Discrete-Time Integrator : DiscreteIntegrator  ExternalReset=rising  SampleTime=Ts  LimitOutput=on  UpperSaturationLimit=6.1  LowerSaturationLimit=0  ICPrevOutput=DiscIntNeverNeededParam  ICPrevScaledInput=DiscIntNeverNeededParam
  Logical Operator1 : Logic  Operator=OR
  Relational Operator3 : RelationalOperator  Operator=>
  Relational Operator4 : RelationalOperator  Operator=>
  Relational Operator5 : RelationalOperator  Operator=<
  Select actual Iq Limit : MultiPortSwitch  Inputs=8
  Switch : Switch  Threshold=0.5
  Switch2 : Switch  Threshold=0.5
  Unit Delay : UnitDelay  SampleTime=Ts  HasFrameUpgradeWarning=on
  Unit Delay5 : UnitDelay  InitialCondition=1  SampleTime=Ts  HasFrameUpgradeWarning=on
  IqLimit : Outport  VectorParamsAs1DForOutWhenUnconnected=off
  wires:
  Constant4/1 -> Select actual Iq Limit/7
  Constant5/1 -> Select actual Iq Limit/8
  Constant8/1 -> Select actual Iq Limit/9
  Constant6/1 -> Select actual Iq Limit/2
  Constant7/1 -> Select actual Iq Limit/3
  Constant1/1 -> Select actual Iq Limit/4
  Constant2/1 -> Select actual Iq Limit/5
  Constant3/1 -> Select actual Iq Limit/6
  Select actual Iq Limit/1 -> IqLimit/1
  Logical Operator1/1 -> Switch2/2
  Switch2/1 -> Unit Delay5/1
  Unit Delay5/1 -> Select actual Iq Limit/1, Switch2/3, Relational Operator3/1, Relational Operator5/1
  Relational Operator3/1 -> Switch/2
  Constant10/1 -> Switch/3
  Constant9/1 -> Switch/1
  Unit Delay/1 -> Discrete-Time Integrator/2
  Switch/1 -> Discrete-Time Integrator/1
  Constant11/1 -> Relational Operator4/2
  Discrete-Time Integrator/1 -> Relational Operator4/1
  Relational Operator4/1 -> Unit Delay/1, Logical Operator1/1
  Relational Operator5/1 -> Logical Operator1/2
  IqLimit_Index/1 -> Switch2/1, Relational Operator3/2, Relational Operator5/2

== system STATCOM/STATCOM Controller/Measurement System/Mean value ==
  note: Variable frequency - Discrete Mean Value
  note: Pierre Giroux, Gilbert Sybille
      | Power System Simulation Laboratory
      | IREQ, Hydro-Quebc
  Freq : Inport
  In : Inport  Port=2
  Constant : Constant  Value=Vinit
  Gain : Gain  Gain=Ts  SaturateOnIntegerOverflow=on  OutDataTypeStr=Inherit: Same as input  ParamDataTypeStr=Inherit: Same as input
  Integ4 : DiscreteIntegrator  IntegratorMethod=Integration: Trapezoidal  SampleTime=Ts  ICPrevOutput=DiscIntNeverNeededParam  ICPrevScaledInput=DiscIntNeverNeededParam
  K2 : Constant  Value=Ts/2
  Number of sample/cycle : Fcn  Expr=1/(u[1]+1e-6)/Ts
  Product : Product  InputSameDT=on  SaturateOnIntegerOverflow=on  OutDataTypeStr=Inherit: Same as first input
  Product1 : Product  Inputs=*/*  InputSameDT=on  SaturateOnIntegerOverflow=on  OutDataTypeStr=Inherit: Same as first input
  Rounding Function : Rounding  Operator=round
  Step : Step  Time=1/Finit  SampleTime=Ts
  Sum3 : Sum  Inputs=-+  InputSameDT=on  SaturateOnIntegerOverflow=on  OutDataTypeStr=Inherit: Same as first input
  Sum4 : Sum  Inputs=-+  InputSameDT=on  SaturateOnIntegerOverflow=on  OutDataTypeStr=Inherit: Same as first input
  Sum5 : Sum  InputSameDT=on  SaturateOnIntegerOverflow=on  OutDataTypeStr=Inherit: Same as first input
  Sum7 : Sum  Inputs=-+  InputSameDT=on  SaturateOnIntegerOverflow=on  OutDataTypeStr=Inherit: Same as first input
  Switch : Switch  Threshold=0.5
  Variable Transport Delay2 : VariableTransportDelay  MaximumDelay=20e-3
  Mean : Outport  VectorParamsAs1DForOutWhenUnconnected=off
  wires:
  Switch/1 -> Mean/1
  Constant/1 -> Switch/3
  Step/1 -> Switch/2
  Sum5/1 -> Switch/1
  Sum3/1 -> Variable Transport Delay2/2  "Delay"
  Number of sample/cycle/1 -> Sum4/2, Rounding Function/1
  Sum4/1 -> Product1/1
  Rounding Function/1 -> Sum4/1, Product1/2, Gain/1
  Gain/1 -> Sum3/2
  K2/1 -> Sum3/1
  Freq/1 -> Number of sample/cycle/1, Product/2  "Freq"
  Integ4/1 -> Sum7/2, Variable Transport Delay2/1
  Sum7/1 -> Product/1
  Variable Transport Delay2/1 -> Sum7/1
  Product/1 -> Sum5/1  "Mean value"
  In/1 -> Integ4/1, Product1/3  "In"
  Product1/1 -> Sum5/2  "Correction"

== system STATCOM/STATCOM Controller/Measurement System/PQ Computaion ==
  note: PQ Measurement:
  note: Q = Vq*Id-Vd*Iq
  note: P = Vd*Id + Vq*Iq
  Vd_Vq : Inport  PortDimensions=2
  Id_Iq : Inport  Port=2  PortDimensions=2
  Freq : Inport  Port=3  PortDimensions=1
  Demux1 : Demux  Outputs=2
      settings: DisplayOption=none
  Demux2 : Demux  Outputs=2
      settings: DisplayOption=none
  Mux2 : Mux  Inputs=2
  Product{2..5} (4 alike) : Product  InputSameDT=on  SaturateOnIntegerOverflow=on  OutDataTypeStr=Inherit: Same as first input
  Sum : Sum  InputSameDT=on  SaturateOnIntegerOverflow=on  OutDataTypeStr=Inherit: Same as first input
  Sum1 : Sum  Inputs=+-  InputSameDT=on  SaturateOnIntegerOverflow=on  OutDataTypeStr=Inherit: Same as first input
  Variable Frequency Mean value : Subsystem  mask(Discrete Variable-Frequency Mean Value){Finit=60, Vinit=0, Ts=Ts}
      mask prompts: Finit "Initial Frequency (Hz):"; Vinit "Initial input (DC component):"; Ts "Sample time:"
      mask help:
      | This discrete block computes the mean value of the input signal (port In) over a running window of one cycle of a specified frequency (port Freq).
      |
      | For the first cycle of simulation (specified by the parameter "Initial frequency"), the output is held to the value of the  "Initial input" parameter.
  PQ(pu) : Outport  VectorParamsAs1DForOutWhenUnconnected=off
  wires:
  Vd_Vq/1 -> Demux1/1
  Id_Iq/1 -> Demux2/1
  Freq/1 -> Variable Frequency Mean value/1(Freq)
  Variable Frequency Mean value/1(Mean) -> PQ(pu)/1
  Mux2/1 -> Variable Frequency Mean value/2(In)
  Demux2/2 -> Product5/2, Product3/2
  Demux1/1 -> Product5/1, Product2/1
  Demux2/1 -> Product4/2, Product2/2
  Demux1/2 -> Product4/1, Product3/1
  Sum1/1 -> Mux2/2
  Sum/1 -> Mux2/1
  Product5/1 -> Sum1/2
  Product4/1 -> Sum1/1
  Product3/1 -> Sum/2
  Product2/1 -> Sum/1

== system STATCOM/STATCOM Controller/Measurement System/Reactive current measurement (Iq) ==
  note: Vq= 2/3 (Va*coswt + Vb*cos(wt-2pi/3) + Vc*cos(wt+2pi/3)
  note: cos
  note: cos
  note: sin
  note: Vd= 2/3 (Va*sinwt + Vb*sin(wt-2pi/3) + Vc*sin(wt+2pi/3)
  note: V0= 1/3 (Va + Vb + Vc )
  sin_cos : Inport
  abc : Inport  Port=2
  Demux : Demux  Outputs=2
      settings: DisplayOption=none
  Fcn1 : Fcn  Expr=2/3*((u[1]*u[5])+(u[2]*u[7])+(u[3]*u[9]))
  Fcn2 : Fcn  Expr=2/3*((u[1]*u[4])+(u[2]*u[6])+(u[3]*u[8]))
  K1 : Constant  Value=0.5
  K2 : Constant  Value=sqrt(3)/2
  Mux : Mux  Inputs=2
  Mux1 : Mux  Inputs=2
  Mux2 : Mux  Inputs=6
  Product{,1..3} (4 alike) : Product  InputSameDT=on  SaturateOnIntegerOverflow=on  OutDataTypeStr=Inherit: Same as first input
  Sum : Sum  Inputs=--  InputSameDT=on  SaturateOnIntegerOverflow=on  OutDataTypeStr=Inherit: Same as first input
  Sum1 : Sum  Inputs=-+  InputSameDT=on  SaturateOnIntegerOverflow=on  OutDataTypeStr=Inherit: Same as first input
  Sum2 : Sum  Inputs=--  InputSameDT=on  SaturateOnIntegerOverflow=on  OutDataTypeStr=Inherit: Same as first input
  Sum3 : Sum  Inputs=--  InputSameDT=on  SaturateOnIntegerOverflow=on  OutDataTypeStr=Inherit: Same as first input
  IdIq : Outport  InitialOutput=0  VectorParamsAs1DForOutWhenUnconnected=off
  wires:
  Mux1/1 -> IdIq/1
  Fcn1/1 -> Mux1/2  "Iq"
  Fcn2/1 -> Mux1/1  "Id"
  Mux/1 -> Fcn2/1, Fcn1/1
  abc/1 -> Mux/1  "Vabc"
  Mux2/1 -> Mux/2
  sin_cos/1 -> Demux/1
  Demux/2 -> Sum3/2, Product3/1, Product1/1, Mux2/2  "cos(wt)"
  Demux/1 -> Product/1, Product2/1, Sum2/2, Mux2/1  "sin(wt)"
  Product/1 -> Sum/1
  Product1/1 -> Sum/2
  Product3/1 -> Sum1/1
  Product2/1 -> Sum1/2
  Sum3/1 -> Mux2/6  "cos(wt+2pi/3)"
  Sum2/1 -> Mux2/5  "sin(wt+2pi/3)"
  K1/1 -> Product/2, Product3/2
  K2/1 -> Product1/2, Product2/2
  Sum/1 -> Mux2/3, Sum2/1  "sin(wt-2pi/3)"
  Sum1/1 -> Mux2/4, Sum3/1  "cos(wt-2pi/3)"

== system STATCOM/STATCOM Controller/Measurement System/Voltage measurement (Positive sequence) ==
  note: Pierre Giroux, Gilbert Sybille
      | Power System Simulation Laboratory
      | IREQ, Hydro-Quebc
  note: Discrete 3-phase PLL-Driven Positive-Sequence Fundamental Value
  abc : Inport  PortDimensions=3
  Freq : Inport  Port=2
  wt : Inport  Port=3  PortDimensions=1
  Demux : Demux  Outputs=3
      settings: DisplayOption=none
  Discrete Variable Frequency Mean value1 : Subsystem  mask(Discrete Variable-Frequency Mean Value){Finit=Finit, Vinit=Real_Init, Ts=Ts}
      mask prompts: Finit "Initial Frequency (Hz):"; Vinit "Initial input (DC component):"; Ts "Sample time:"
      mask help:
      | This discrete block computes the mean value of the input signal (port In) over a running window of one cycle of a specified frequency (port Freq).
      |
      | For the first cycle of simulation (specified by the parameter "Initial frequency"), the output is held to the value of the  "Initial input" parameter.
  Discrete Variable Frequency Mean value2 : Subsystem  mask(Discrete Variable-Frequency Mean Value){Finit=Finit, Vinit=Imag_Init, Ts=Ts}
      mask prompts: Finit "Initial Frequency (Hz):"; Vinit "Initial input (DC component):"; Ts "Sample time:"
      mask help:
      | This discrete block computes the mean value of the input signal (port In) over a running window of one cycle of a specified frequency (port Freq).
      |
      | For the first cycle of simulation (specified by the parameter "Initial frequency"), the output is held to the value of the  "Initial input" parameter.
  Fcn3 : Fcn  Expr=sqrt(u[1]*u[1]+u[2]*u[2])
  Mux1 : Mux  Inputs=2
  Selector : Selector  InputPortWidth=3  IndexOptions=Index vector (dialog)  Indices=[1 2]  OutputSizes=1
  Terminator : Terminator
  abc to dq0 : spsabctodq0Lib/abc to dq0  Alignment=90 degrees behind phase A axis
  Mag : Outport  VectorParamsAs1DForOutWhenUnconnected=off
  VdVq : Outport  Port=2  VectorParamsAs1DForOutWhenUnconnected=off
  wires:
  Mux1/1 -> Fcn3/1
  Selector/1 -> VdVq/1
  abc to dq0/1 -> Selector/1, Demux/1
  wt/1 -> abc to dq0/2
  Freq/1 -> Discrete Variable Frequency Mean value2/1(Freq), Discrete Variable Frequency Mean value1/1(Freq)
  Discrete Variable Frequency Mean value1/1(Mean) -> Mux1/1  "Real"
  Fcn3/1 -> Mag/1
  Discrete Variable Frequency Mean value2/1(Mean) -> Mux1/2  "Real"
  Demux/2 -> Discrete Variable Frequency Mean value2/2(In)
  Demux/1 -> Discrete Variable Frequency Mean value1/2(In)
  abc/1 -> abc to dq0/1
  Demux/3 -> Terminator/1
